simulink model "EO_Kalman_LOS_Estimation"  (R2026a)
settings: Solver=FixedStepDiscrete  StopTime=60  FixedStep=0.02
settings Model: Creator=Avatec  LastModifiedBy=Avatec

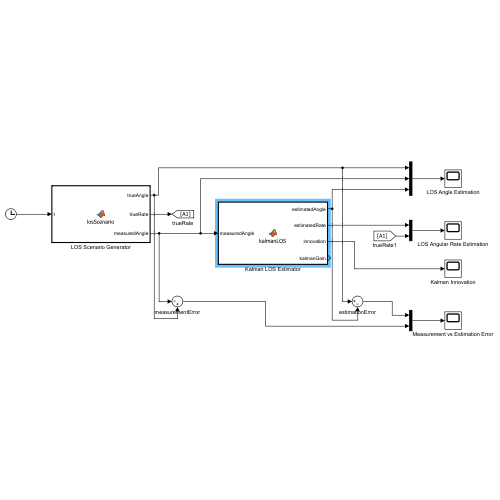
[thumbnail: Simulink's stored preview of the top-level diagram]
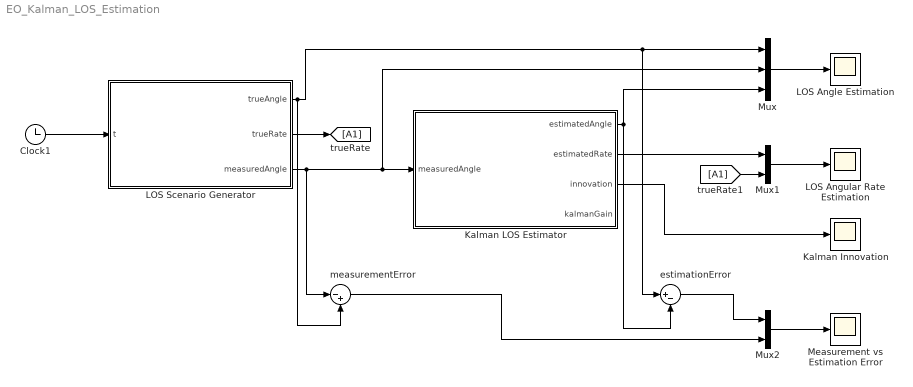
== system EO_Kalman_LOS_Estimation ==
  Clock1 : Clock
  Kalman Innovation : Scope
      settings: ActiveDisplayYMinimum=-5.650138723540417  ActiveDisplayYMaximum=4.012977099791927  DataLoggingVariableName=ScopeData2
  Kalman LOS Estimator : MATLAB Function  TreatAsAtomicUnit=on
  LOS Angle Estimation : Scope
      settings: ActiveDisplayYMinimum=1.9987642607557605  ActiveDisplayYMaximum=8.6706949419586152
  LOS Angular Rate Estimation : Scope
      settings: ActiveDisplayYMinimum=-1.5443244937625096  ActiveDisplayYMaximum=3.2628813515299697
  LOS Scenario Generator : MATLAB Function  TreatAsAtomicUnit=on
  Measurement vs Estimation Error : Scope
      settings: ActiveDisplayYMinimum=-0.56734268301464619  ActiveDisplayYMaximum=0.90731151600857163  DataLoggingVariableName=ScopeData3
  Mux : Mux  Inputs=3
  Mux1 : Mux  Inputs=2
  Mux2 : Mux  Inputs=2
  estimationError : Sum  Inputs=|+-
  measurementError : Sum  Inputs=|-+
  wires:
  Clock1/1 -> LOS Scenario Generator/1(t)
  LOS Scenario Generator/3(measuredAngle) -> measurementError/1, Mux/2, Kalman LOS Estimator/1(measuredAngle)
  Kalman LOS Estimator/1(estimatedAngle) -> estimationError/2, Mux/3
  Mux/1 -> LOS Angle Estimation/1
  Kalman LOS Estimator/2(estimatedRate) -> Mux1/1
  LOS Scenario Generator/2(trueRate) -> [A1]
  [A1] -> Mux1/2
  Mux1/1 -> LOS Angular Rate Estimation/1
  Kalman LOS Estimator/3(innovation) -> Kalman Innovation/1
  LOS Scenario Generator/1(trueAngle) -> estimationError/1, Mux/1, measurementError/2
  estimationError/1 -> Mux2/1
  measurementError/1 -> Mux2/2
  Mux2/1 -> Measurement vs Estimation Error/1

== matlab function EO_Kalman_LOS_Estimation/Kalman LOS Estimator ==
  data: measuredAngle input; estimatedAngle output; estimatedRate output; innovation output; kalmanGain output
function [estimatedAngle, estimatedRate, innovation, kalmanGain] = ...
    kalmanLOS(measuredAngle)

% =========================================================
% 1D CONSTANT VELOCITY KALMAN FILTER
%
% State:
%
% x(1) = LOS angle        [deg]
% x(2) = LOS angular rate [deg/s]
% =========================================================


% ---------------------------------------------------------
% SAMPLE TIME
% ---------------------------------------------------------

Ts = 0.02;


% ---------------------------------------------------------
% PERSISTENT STATES
% ---------------------------------------------------------

persistent x
persistent P


% ---------------------------------------------------------
% INITIALIZATION
% ---------------------------------------------------------

if isempty(x)

    x = [0; 0];

    P = [4 0;
         0 4];

end


% =========================================================
% SYSTEM MODEL
% =========================================================

A = [1 Ts;
     0 1];

H = [1 0];


% ---------------------------------------------------------
% PROCESS NOISE
% ---------------------------------------------------------

Q = [0.001  0;
     0      0.03];


% ---------------------------------------------------------
% MEASUREMENT NOISE VARIANCE
% ---------------------------------------------------------

R = 0.5;


% =========================================================
% PREDICTION
% =========================================================

xPred = A*x;

PPred = A*P*A' + Q;


% =========================================================
% MEASUREMENT UPDATE
% =========================================================

innovation = ...
    measuredAngle - H*xPred;


S = ...
    H*PPred*H' + R;


K = ...
    PPred*H' / S;


x = ...
    xPred + K*innovation;


I = eye(2);

P = ...
    (I - K*H)*PPred;


% =========================================================
% OUTPUTS
% =========================================================

estimatedAngle = x(1);

estimatedRate = x(2);

kalmanGain = K(1);

end

== matlab function EO_Kalman_LOS_Estimation/LOS Scenario Generator ==
  data: t input; trueAngle output; trueRate output; measuredAngle output
function [trueAngle, trueRate, measuredAngle] = losScenario(t)

% =========================================================
% EO LINE-OF-SIGHT TEST SCENARIO
%
% trueAngle     = Actual target LOS angle [deg]
% trueRate      = Actual angular rate [deg/s]
% measuredAngle = Noisy camera measurement [deg]
% =========================================================


% ---------------------------------------------------------
% TRUE TARGET ANGLE
% ---------------------------------------------------------

trueAngle = ...
      5.0*sin(0.35*t) ...
    + 2.5*sin(0.11*t + 0.8) ...
    + 1.2*sin(0.75*t);


% ---------------------------------------------------------
% TRUE ANGULAR RATE
%
% Analytical derivative of trueAngle
% ---------------------------------------------------------

trueRate = ...
      5.0*0.35*cos(0.35*t) ...
    + 2.5*0.11*cos(0.11*t + 0.8) ...
    + 1.2*0.75*cos(0.75*t);


% ---------------------------------------------------------
% CAMERA / SENSOR MEASUREMENT NOISE
% ---------------------------------------------------------

noise = ...
      0.45*sin(13.7*t) ...
    + 0.22*sin(29.3*t + 1.1) ...
    + 0.12*sin(47.5*t + 0.4);


% ---------------------------------------------------------
% SHORT SENSOR DISTURBANCES
% ---------------------------------------------------------

glitch1 = 0.8 * exp(-((t-18)/0.12)^2);

glitch2 = -1.0 * exp(-((t-37)/0.10)^2);

glitch3 = 0.7 * exp(-((t-51)/0.15)^2);


% ---------------------------------------------------------
% CAMERA MEASUREMENT
% ---------------------------------------------------------

measuredAngle = ...
    trueAngle ...
    + noise ...
    + glitch1 ...
    + glitch2 ...
    + glitch3;

end
